simulink model "Bicycle_Model_2020a"  (R2020a)
settings: Solver=ode4  StartTime=0.0  StopTime=30  FixedStep=1e-3  RelTol=1e-3
values from neighbouring files (symbols this model uses):
  Ts = 0.01    [HW03_run_bicycle.m]    (also in HW03_run_kinematic.m)
undefined symbols (not defined in the file or in its folder): data, init, input
libraries: simulink x1
settings Model: Creator=nishantc  LastModifiedBy=Linxi Ren
settings DataIOCC: ReturnWorkspaceOutputs=off
settings DebuggingCC: ArithmeticOperatorsInVariantConditions=warning
settings SFSimCC: CustomCodeUndefinedFunction=UseInterfaceOnly

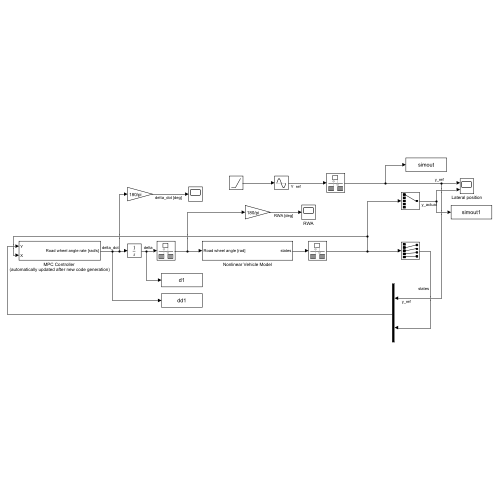
[thumbnail: Simulink's stored preview of the top-level diagram]
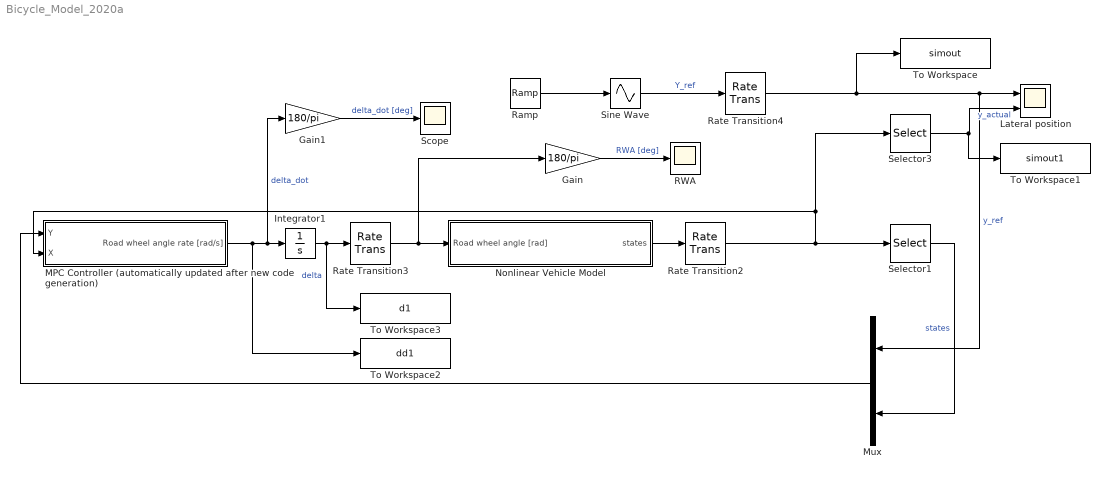
== system Bicycle_Model_2020a ==
  Gain : Gain  Gain=180/pi
  Gain1 : Gain  Gain=180/pi
  Integrator1 : Integrator
  Lateral position : Scope  NumInputPorts=2
  MPC Controller (automatically updated after new code generation) : Subsystem
  Mux : Mux  Inputs=2
  Nonlinear Vehicle Model : Subsystem
  RWA : Scope
  Ramp : simulink/Sources/Ramp  slope=1  start=5  InitialOutput=0
  Rate Transition2 : RateTransition  OutPortSampleTime=Ts
  Rate Transition3 : RateTransition
  Rate Transition4 : RateTransition  OutPortSampleTime=Ts
  Scope : Scope
  Selector1 : Selector  InputPortWidth=5  IndexOptions=Index vector (dialog)  Indices=[2:5]  OutputSizes=1
  Selector3 : Selector  InputPortWidth=5  IndexOptions=Index vector (dialog)  Indices=1  OutputSizes=1
  Sine Wave : Sin  TimeSource=Use external signal  Frequency=2*pi*0.2  SampleTime=0
  To Workspace : ToWorkspace  VariableName=simout  SaveFormat=Timeseries  SampleTime=-1
  To Workspace1 : ToWorkspace  VariableName=simout1  SaveFormat=Timeseries  SampleTime=-1
  To Workspace2 : ToWorkspace  VariableName=dd1  SaveFormat=Timeseries  SampleTime=-1
  To Workspace3 : ToWorkspace  VariableName=d1  SaveFormat=Timeseries  SampleTime=-1
  wires:
  MPC Controller (automatically updated after new code generation)/1(Road wheel angle rate [rad/s]) -> To Workspace2/1, Gain1/1, Integrator1/1  "delta_dot"
  Mux/1 -> MPC Controller (automatically updated after new code generation)/1(Y)
  Ramp/1 -> Sine Wave/1
  Nonlinear Vehicle Model/1(states) -> Rate Transition2/1
  Selector1/1 -> Mux/2  "states"
  Selector3/1 -> To Workspace1/1, Lateral position/2  "y_actual"
  Rate Transition4/1 -> To Workspace/1, Mux/1, Lateral position/1  "y_ref"
  Rate Transition2/1 -> Selector3/1, MPC Controller (automatically updated after new code generation)/2(X), Selector1/1
  Sine Wave/1 -> Rate Transition4/1  "Y_ref"
  Integrator1/1 -> To Workspace3/1, Rate Transition3/1  "delta"
  Gain/1 -> RWA/1  "RWA [deg]"
  Rate Transition3/1 -> Nonlinear Vehicle Model/1(Road wheel angle [rad]), Gain/1
  Gain1/1 -> Scope/1  "delta_dot [deg]"

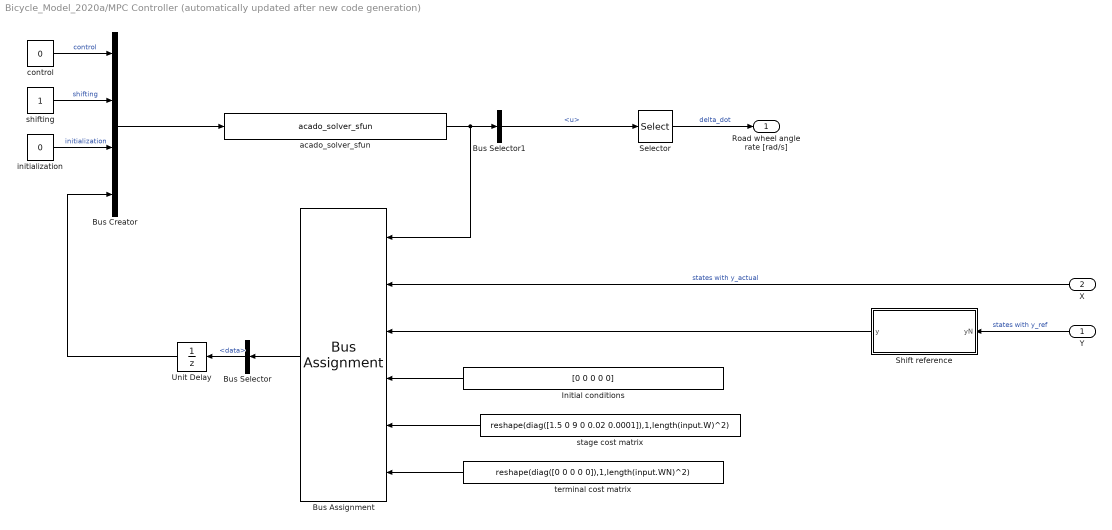
== system Bicycle_Model_2020a/MPC Controller (automatically updated after new code generation) ==
  Y : Inport
  X : Inport  Port=2
  Bus Assignment : BusAssignment  AssignedSignals=data.x0,data.y,data.yN,data.W,data.WN
  Bus Creator : BusCreator  Inputs=4  OutDataTypeStr=Bus: ACADOinput
  Bus Selector : BusSelector  OutputSignals=data
  Bus Selector1 : BusSelector  OutputSignals=data.u
  Initial conditions : Constant  Value=[0 0 0 0 0]
  Selector : Selector  InputPortWidth=Np  IndexOptions=Starting index (dialog)  Indices=[1]  OutputSizes=1
  Shift reference : MATLAB Function  TreatAsAtomicUnit=on
  Unit Delay : UnitDelay  InitialCondition=init  SampleTime=Ts  HasFrameUpgradeWarning=on
  acado_solver_sfun : S-Function  FunctionName=acado_solver_sfun  SFunctionDeploymentMode=off  EnableBusSupport=off  mask(Legacy Function){SFunctionSpec=acado_step(ACADOinput u1[1], ACADOoutput y1[1]), ShowSpec=on}
      mask prompts: ShowSpec "Display function specification"
      mask help:
      | This block allows you to call the legacy functions specified by the following Legacy Code Tool definition:
      | def.SFunctionName = 'acado_solver_sfun';
      | def.OutputFcnSpec = 'acado_step(ACADOinput u1[1], ACADOoutput y1[1])';
      | def.StartFcnSpec = 'acado_initialize( void )';
      | def.TerminateFcnSpec = 'acado_cleanup( void )';
      | def.HeaderFiles = {'acado_common.h', 'acado_solver_sfunction.h'};
      | def.SourceFiles = {'acado_solver.c', 'acado_integrator.c', 'acado_auxiliary_functions.c', 'acado_solver_sfunction.c', 'acado_qpoases3_interface.c', 'qpoases3\src\Bounds.c', 'qpoases3\src\Constraints.c', 'qpoases3\src\Indexlist.c', 'qpoases3\src\Matrices.c', 'qpoases3\src\MessageHandling.c', 'qpoases3\src\Options.c', 'qpoases3\src\Flipper.c', 'qpoases3\src\QProblem.c', 'qpoases3\src\QProblemB.c', 'qpoases3\src\Utils.c'};
      mask Help: <p>This block was generated automatically by the Legacy Code Tool. For detailed help on this tool, call<a href="matlab:legacy_code('help')"> legacy_code('help')</a>.</p>
      mask Callback ShowSpec:
      | if strcmp(get_param(gcbh, 'ShowSpec'), 'on')
      |   set_param(gcbh, 'MaskDisplay', sprintf('fprintf(''%s'');', get_param(gcbh, 'SFunctionSpec')));
      | else
      |   set_param(gcbh, 'MaskDisplay', sprintf('fprintf(''%s'');', get_param(gcbh, 'FunctionName')));
      | end
      mask Display: fprintf('acado_step(ACADOinput u1[1], ACADOoutput y1[1])');
  control : Constant  Value=0  OutDataTypeStr=int32
  initialization : Constant  Value=0  OutDataTypeStr=int32
  shifting : Constant  OutDataTypeStr=int32
  stage cost matrix : Constant  Value=reshape(diag([1.5 0 9 0 0.02 0.0001]),1,length(input.W)^2)
  terminal cost matrix : Constant  Value=reshape(diag([0 0 0 0 0]),1,length(input.WN)^2)
  Road wheel angle rate [rad/s] : Outport
  wires:
  control/1 -> Bus Creator/1  "control"
  Bus Selector1/1 -> Selector/1  "<u>"
  initialization/1 -> Bus Creator/3  "initialization"
  acado_solver_sfun/1 -> Bus Selector1/1, Bus Assignment/1
  shifting/1 -> Bus Creator/2  "shifting"
  X/1 -> Bus Assignment/2  "states with y_actual"
  Bus Assignment/1 -> Bus Selector/1
  terminal cost matrix/1 -> Bus Assignment/6
  Initial conditions/1 -> Bus Assignment/4
  Shift reference/1(y) -> Bus Assignment/3
  stage cost matrix/1 -> Bus Assignment/5
  Bus Selector/1 -> Unit Delay/1  "<data>"
  Unit Delay/1 -> Bus Creator/4
  Bus Creator/1 -> acado_solver_sfun/1
  Selector/1 -> Road wheel angle rate [rad/s]/1  "delta_dot"
  Y/1 -> Shift reference/1(yN)  "states with y_ref"

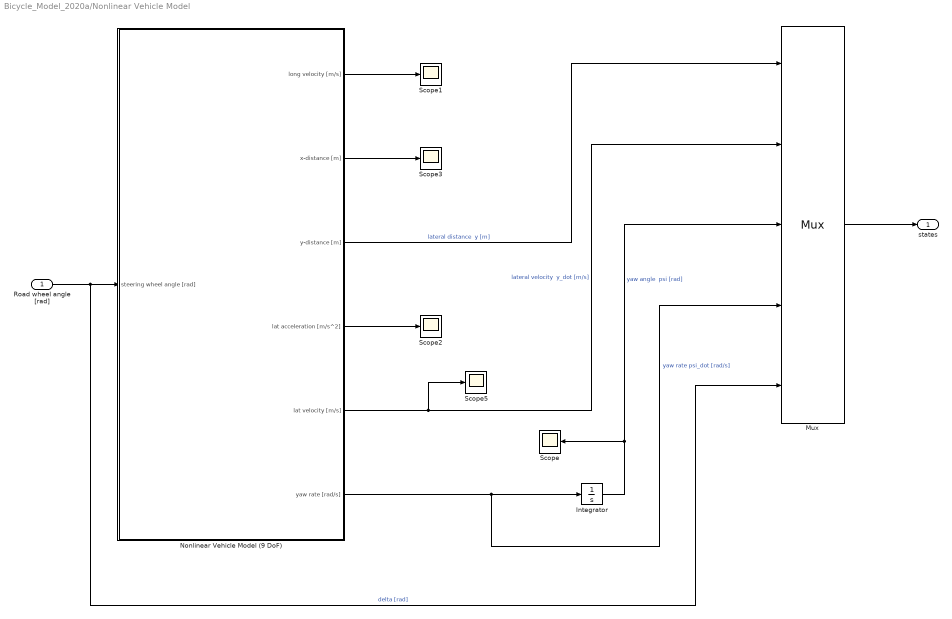
== system Bicycle_Model_2020a/Nonlinear Vehicle Model ==
  Road wheel angle [rad] : Inport
  Integrator : Integrator
  Mux : Mux  Inputs=5
      settings: DisplayOption=signals
  Nonlinear Vehicle Model (9 DoF) : Subsystem
      mask help: Simulink:masks:GenSFuncDesc_MD
      mask Help: eval('feval(''rtwprivate'',''rtwhelpview'',''rtw_sfcn_block'')');
  Scope{,1..3,5} (5 alike) : Scope
  states : Outport  VectorParamsAs1DForOutWhenUnconnected=off
  wires:
  Nonlinear Vehicle Model (9 DoF)/4(lat acceleration [m/s^2]) -> Scope2/1
  Nonlinear Vehicle Model (9 DoF)/5(lat velocity [m/s]) -> Mux/2, Scope5/1  "lateral velocity  y_dot [m/s]"
  Nonlinear Vehicle Model (9 DoF)/6(yaw rate [rad/s]) -> Integrator/1, Mux/4  "yaw rate psi_dot [rad/s]"
  Mux/1 -> states/1
  Nonlinear Vehicle Model (9 DoF)/1(long velocity [m/s]) -> Scope1/1
  Integrator/1 -> Mux/3, Scope/1  "yaw angle  psi [rad]"
  Road wheel angle [rad]/1 -> Mux/5, Nonlinear Vehicle Model (9 DoF)/1(steering wheel angle [rad])  "delta [rad]"
  Nonlinear Vehicle Model (9 DoF)/3(y-distance [m]) -> Mux/1  "lateral distance  y [m]"
  Nonlinear Vehicle Model (9 DoF)/2(x-distance [m]) -> Scope3/1

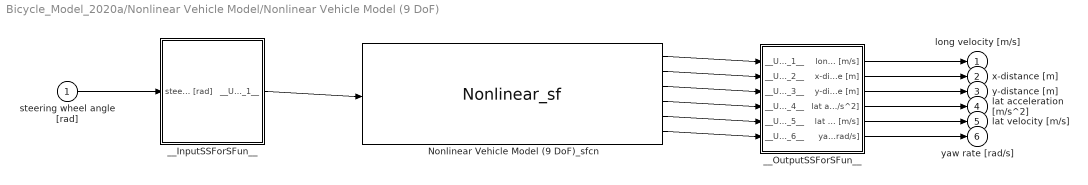
== system Bicycle_Model_2020a/Nonlinear Vehicle Model/Nonlinear Vehicle Model (9 DoF) ==
  steering wheel angle [rad] : Inport
  Nonlinear Vehicle Model (9 DoF)_sfcn : S-Function  FunctionName=Nonlinear_sf  SFunctionModules=""  SFunctionDeploymentMode=off  EnableBusSupport=off  mask{rtw_sf_name=Nonlinear_sf, showVar=off}
      mask prompts: rtw_sf_name "Simulink:masks:GenSFuncName_MP"; showVar "Simulink:masks:GenSFuncShowModuleList_MP"
      mask help: Simulink:masks:GenSFuncDesc_MD
      mask init:
      | displist = '';
      | if ~strcmp(get_param(gcb, 'FunctionName'), rtw_sf_name);
      |   set_param(gcb, 'FunctionName', rtw_sf_name);
      | end
      | % Check if we are generating code
      | rtw_mode = false;
      | if strcmpi(get_param(bdroot(gcb),'SimulationStatus'),'Initializing')
      | 	rtw_mode = strcmpi(get_param(bdroot(gcb),'BuildingRTWCode'),'on') && ...
      | 		~strcmpi(get_param(bdroot(gcb),'TargetStyle'),'SimulationTarget');
      | end
      | if showVar || rtw_mode
      | 	if exist('rtwsfunc') == 2 | exist('rtwsfunc') == 6
      | 		tmplist = rtwsfunc(rtw_sf_name,gcb);
      | 		tmplist = DAStudio.message('Simulink:masks:GenSFuncListOfModules_IC', tmplist);
      | 	elseif showVar
      | 		tmplist1 = DAStudio.message('Simulink:masks:GenSFuncListOfModules_IC', '');
      |         tmplist2 = DAStudio.message('Simulink:masks:GenSFuncNotLicensed_IC');
      |         tmplist = [tmplist1 tmplist2];
      |  	end
      | end
      | if showVar
      |   displist = tmplist;
      | end
      settings: CopyFcn=|
      | if ~strcmp(get_param(gcb,'Linkstatus'),'none') && ...
      | ~strcmp(get_param(gcb,'Linkstatus'),'implicit')
      |   set_param(gcb,'LinkStatus','none');
      | end
      mask Help: eval('feval(''rtwprivate'',''rtwhelpview'',''rtw_sfcn_block'')');
      mask Display:
      | port_label('input',1,'steering wheel angle [rad]');
      | port_label('output',1,'long velocity [m/s]');
      | port_label('output',2,'x-distance [m]');
      | port_label('output',3,'y-distance [m]');
      | port_label('output',4,'lat acceleration [m/s^2]');
      | port_label('output',5,'lat velocity [m/s]');
      | port_label('output',6,'yaw rate [rad/s]');
  __InputSSForSFun__ : Subsystem
  __OutputSSForSFun__ : Subsystem
  long velocity [m/s] : Outport  VectorParamsAs1DForOutWhenUnconnected=off
  x-distance [m] : Outport  Port=2  VectorParamsAs1DForOutWhenUnconnected=off
  y-distance [m] : Outport  Port=3  VectorParamsAs1DForOutWhenUnconnected=off
  lat acceleration [m/s^2] : Outport  Port=4  VectorParamsAs1DForOutWhenUnconnected=off
  lat velocity [m/s] : Outport  Port=5  VectorParamsAs1DForOutWhenUnconnected=off
  yaw rate [rad/s] : Outport  Port=6  VectorParamsAs1DForOutWhenUnconnected=off
  wires:
  steering wheel angle [rad]/1 -> __InputSSForSFun__/1(steering wheel angle [rad])
  __InputSSForSFun__/1(__UniqueOutportName__1__) -> Nonlinear Vehicle Model (9 DoF)_sfcn/1
  Nonlinear Vehicle Model (9 DoF)_sfcn/1 -> __OutputSSForSFun__/1(__UniqueInportName__1__)
  Nonlinear Vehicle Model (9 DoF)_sfcn/2 -> __OutputSSForSFun__/2(__UniqueInportName__2__)
  Nonlinear Vehicle Model (9 DoF)_sfcn/3 -> __OutputSSForSFun__/3(__UniqueInportName__3__)
  Nonlinear Vehicle Model (9 DoF)_sfcn/4 -> __OutputSSForSFun__/4(__UniqueInportName__4__)
  Nonlinear Vehicle Model (9 DoF)_sfcn/5 -> __OutputSSForSFun__/5(__UniqueInportName__5__)
  Nonlinear Vehicle Model (9 DoF)_sfcn/6 -> __OutputSSForSFun__/6(__UniqueInportName__6__)
  __OutputSSForSFun__/1(long velocity [m/s]) -> long velocity [m/s]/1
  __OutputSSForSFun__/2(x-distance [m]) -> x-distance [m]/1
  __OutputSSForSFun__/3(y-distance [m]) -> y-distance [m]/1
  __OutputSSForSFun__/4(lat acceleration [m/s^2]) -> lat acceleration [m/s^2]/1
  __OutputSSForSFun__/5(lat velocity [m/s]) -> lat velocity [m/s]/1
  __OutputSSForSFun__/6(yaw rate [rad/s]) -> yaw rate [rad/s]/1

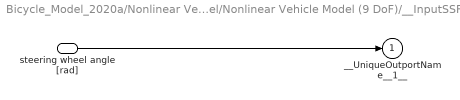
== system Bicycle_Model_2020a/Nonlinear Vehicle Model/Nonlinear Vehicle Model (9 DoF)/__InputSSForSFun__ ==
  steering wheel angle [rad] : Inport
  __UniqueOutportName__1__ : Outport
  wires:
  steering wheel angle [rad]/1 -> __UniqueOutportName__1__/1

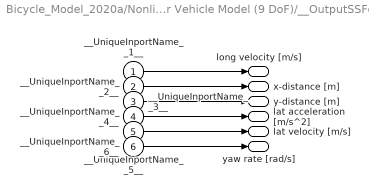
== system Bicycle_Model_2020a/Nonlinear Vehicle Model/Nonlinear Vehicle Model (9 DoF)/__OutputSSForSFun__ ==
  __UniqueInportName__1__ : Inport
  __UniqueInportName__2__ : Inport  Port=2
  __UniqueInportName__3__ : Inport  Port=3
  __UniqueInportName__4__ : Inport  Port=4
  __UniqueInportName__5__ : Inport  Port=5
  __UniqueInportName__6__ : Inport  Port=6
  long velocity [m/s] : Outport  VectorParamsAs1DForOutWhenUnconnected=off
  x-distance [m] : Outport  Port=2  VectorParamsAs1DForOutWhenUnconnected=off
  y-distance [m] : Outport  Port=3  VectorParamsAs1DForOutWhenUnconnected=off
  lat acceleration [m/s^2] : Outport  Port=4  VectorParamsAs1DForOutWhenUnconnected=off
  lat velocity [m/s] : Outport  Port=5  VectorParamsAs1DForOutWhenUnconnected=off
  yaw rate [rad/s] : Outport  Port=6  VectorParamsAs1DForOutWhenUnconnected=off
  wires:
  __UniqueInportName__1__/1 -> long velocity [m/s]/1
  __UniqueInportName__2__/1 -> x-distance [m]/1
  __UniqueInportName__3__/1 -> y-distance [m]/1
  __UniqueInportName__4__/1 -> lat acceleration [m/s^2]/1
  __UniqueInportName__5__/1 -> lat velocity [m/s]/1
  __UniqueInportName__6__/1 -> yaw rate [rad/s]/1

== matlab function Bicycle_Model_2020a/MPC Controller (automatically updated after new code generation)/Shift reference ==
  data: y output; yN input; Np parameter
function y = shift_reference(yN,Np)

y=repmat([yN;0],Np,1)';

end
